simulink model "simulating astronaut"  (R2019b)
settings: Solver=ode45  StartTime=0.0  StopTime=600  FixedStep=.001  MaxStep=.01  MinStep=.001  RelTol=1e-3
values from neighbouring files (symbols this model uses):
  cmw_kPa = 0.0980665    [simulating astronaut.m]
  D = [1e-3 1e-2 0.545e-4]    [simulating astronaut.m]
  dc_metabool = [-0.250 0.200 0]/60    [simulating astronaut.m]
  dV_CO = 5/60    (= 0.0833333333333)    [simulating astronaut.m]
  f_alv_init = [0.154 0.0451 0.79 ]    [simulating astronaut.m]
  f_LW_init = [0.174 0.0291 0.79]    [simulating astronaut.m]
  Hbx_PA_init = [2.44 6.560 ]*1e-3    [simulating astronaut.m]
  Hbx_PC_init = [.564 8.436 ]*1e-3    [simulating astronaut.m]
  Hbx_SA_init = [.520 8.480 ]*1e-3    [simulating astronaut.m]
  Hbx_SC_init = [2.44 6.560 ]*1e-3    [simulating astronaut.m]
  k = 25.45    [simulating astronaut.m]
  P_LWO_EE = 5    [simulating astronaut.m]
  P_LWO_insp = 10    [simulating astronaut.m]
  p_O2_grenswaarde = 16    [simulating astronaut.m]
  p_PA_init = [4.34 11.3 56]    [simulating astronaut.m]
  p_PC_init = [6.92 3.45 55.7]    [simulating astronaut.m]
  p_SA_init = [7.11 3.26 56.4]    [simulating astronaut.m]
  p_SC_init = [4.34 11.3 56]    [simulating astronaut.m]
  p_weefsel_init = [4.33 11.3 56]    [simulating astronaut.m]
  period = 6    [simulating astronaut.m]
  pulse_width = 35    [simulating astronaut.m]
  R = [R_LW R_alv]    [simulating astronaut.m]
  s = [2.4e-4 5e-3 1.23e-4]    [simulating astronaut.m]
  t_left = 10    [simulating astronaut.m]
  t_right = 40    [simulating astronaut.m]
  V_init = [0.82 3.28]    [simulating astronaut.m]
  V_PC = .08    (= 0.08)    [simulating astronaut.m]
  V_SC = 0.250    (= 0.25)    [simulating astronaut.m]
  V_w = 5    [simulating astronaut.m]
  x_alv = [0.001 2 2.75 0.8]    [simulating astronaut.m]
  x_LW = [0.001 8 11 0.2]    [simulating astronaut.m]
  x_TW = [-240 -2.3 5 4.6]    [simulating astronaut.m]
settings Model: Creator=psomhorst  LastModifiedBy=Pruijt
settings DebuggingCC: ArithmeticOperatorsInVariantConditions=warning
settings SFSimCC: CustomCodeUndefinedFunction=UseInterfaceOnly

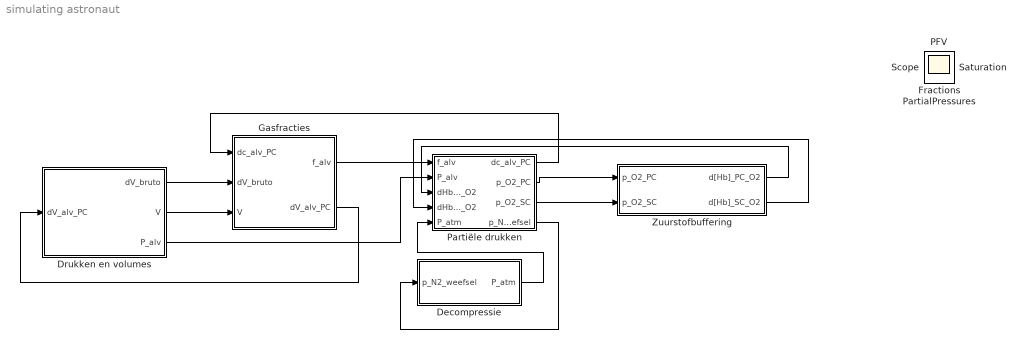
== system simulating astronaut ==
  "Decompressie " : Subsystem
  Drukken en volumes : Subsystem
  Gasfracties : Subsystem
  Partiële drukken : Subsystem
  "Zuurstofbuffering " : Subsystem
  Fractions : Scope
  PFV : Scope
  PartialPressures : Scope
  Saturation : Scope
  Scope : Scope
  wires:
  Drukken en volumes/1(dV_bruto) -> Gasfracties/2(dV_bruto)
  Drukken en volumes/2(V) -> Gasfracties/3(V)
  Gasfracties/2(dV_alv_PC) -> Drukken en volumes/1(dV_alv_PC)
  Gasfracties/1(f_alv) -> Partiële drukken/1(f_alv)
  Drukken en volumes/3(P_alv) -> Partiële drukken/2(P_alv)
  Partiële drukken/1(dc_alv_PC) -> Gasfracties/1(dc_alv_PC)
  Partiële drukken/2(p_O2_PC) -> "Zuurstofbuffering "/1(p_O2_PC)
  "Zuurstofbuffering "/1(d[Hb]_PC_O2) -> Partiële drukken/3(dHb_PC_O2)
  "Zuurstofbuffering "/2(d[Hb]_SC_O2) -> Partiële drukken/4(dHb_SC_O2)
  "Decompressie "/1("P_atm ") -> Partiële drukken/5("P_atm ")
  Partiële drukken/4("p_N2_weefsel ") -> "Decompressie "/1("p_N2_weefsel ")
  Partiële drukken/3(p_O2_SC) -> "Zuurstofbuffering "/2(p_O2_SC)

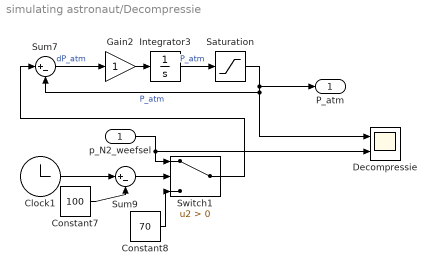
== system simulating astronaut/Decompressie  ==
  "p_N2_weefsel " : Inport
  Clock1 : Clock
  Constant7 : Constant  Value=100
  Constant8 : Constant  Value=70
  "Decompressie " : Scope  NumInputPorts=2
  Gain2 : Gain
  Integrator3 : Integrator  InitialCondition=70
  Saturation : Saturate  UpperLimit=71  LowerLimit=30
  Sum7 : Sum  Inputs=|+-
  Sum9 : Sum  Inputs=|+-
  Switch1 : Switch  Criteria=u2 > Threshold
  "P_atm " : Outport
  wires:
  Gain2/1 -> Integrator3/1
  Sum7/1 -> Gain2/1  "dP_atm"
  Integrator3/1 -> Saturation/1  "P_atm"
  Saturation/1 -> "Decompressie "/1, Sum7/2, "P_atm "/1  "P_atm"
  Constant7/1 -> Sum9/2
  Clock1/1 -> Sum9/1
  Sum9/1 -> Switch1/2
  "p_N2_weefsel "/1 -> "Decompressie "/2, Switch1/1
  Constant8/1 -> Switch1/3
  Switch1/1 -> Sum7/1

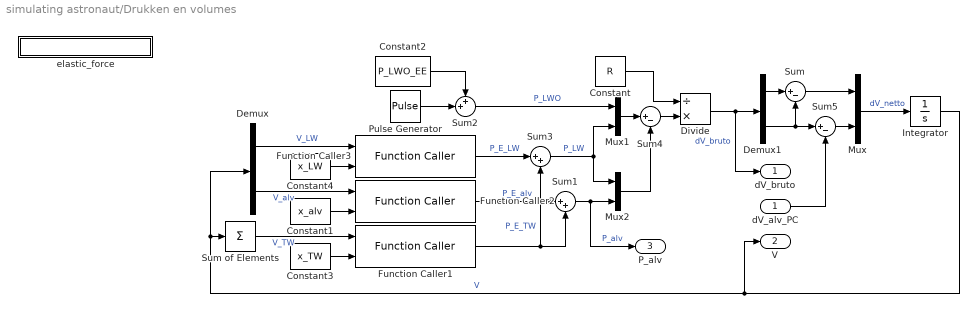
== system simulating astronaut/Drukken en volumes ==
  dV_alv_PC : Inport
  Constant : Constant  Value=R
  Constant1 : Constant  Value=x_alv
  Constant2 : Constant  Value=P_LWO_EE
  Constant3 : Constant  Value=x_TW
  Constant4 : Constant  Value=x_LW
  Demux : Demux  Outputs=2
  Demux1 : Demux  Outputs=2
  Divide : Product  Inputs=/*
  Function Caller1 : FunctionCaller  FunctionPrototype=P_E = elastic_force(V,x)  InputArgumentSpecifications=<Enter example>  OutputArgumentSpecifications=<Enter example>
  Function Caller2 : FunctionCaller  FunctionPrototype=P_E = elastic_force(V,x)  InputArgumentSpecifications=<Enter example>  OutputArgumentSpecifications=<Enter example>
  Function Caller3 : FunctionCaller  FunctionPrototype=P_E = elastic_force(V,x)  InputArgumentSpecifications=<Enter example>  OutputArgumentSpecifications=<Enter example>
  Integrator : Integrator  InitialCondition=V_init
  Mux : Mux  Inputs=2
  Mux1 : Mux  Inputs=2
  Mux2 : Mux  Inputs=2
  Pulse Generator : DiscretePulseGenerator  PulseType=Time based  Amplitude=P_LWO_insp  Period=period  PulseWidth=pulse_width
  Sum : Sum  Inputs=|+-
  Sum of Elements : Sum  Inputs=+
  Sum1 : Sum  Inputs=|++
  Sum2 : Sum  Inputs=++|
  Sum3 : Sum  Inputs=|++
  Sum4 : Sum  Inputs=|+-
  Sum5 : Sum  Inputs=|+-
  elastic_force : Subsystem  TreatAsAtomicUnit=on
  dV_bruto : Outport
  V : Outport  Port=2
  P_alv : Outport  Port=3
  wires:
  Mux2/1 -> Sum4/2
  Sum1/1 -> P_alv/1, Mux2/2  "P_alv"
  Demux/1 -> Function Caller3/1  "V_LW"
  Sum2/1 -> Mux1/1  "P_LWO"
  Mux1/1 -> Sum4/1
  Sum3/1 -> Mux2/1, Mux1/2  "P_LW"
  Demux1/1 -> Sum/1
  Function Caller3/1 -> Sum3/1  "P_E_LW"
  Function Caller2/1 -> Sum1/1  "P_E_alv"
  Sum of Elements/1 -> Function Caller1/1  "V_TW"
  Constant2/1 -> Sum2/1
  Pulse Generator/1 -> Sum2/2
  Constant4/1 -> Function Caller3/2
  Divide/1 -> Demux1/1, dV_bruto/1  "dV_bruto"
  Demux/2 -> Function Caller2/1  "V_alv"
  Integrator/1 -> Demux/1, Sum of Elements/1, V/1  "V"
  Sum/1 -> Mux/1
  Sum4/1 -> Divide/2
  Mux/1 -> Integrator/1  "dV_netto"
  Function Caller1/1 -> Sum1/2, Sum3/2  "P_E_TW"
  Constant1/1 -> Function Caller2/2
  Constant3/1 -> Function Caller1/2
  Demux1/2 -> Sum5/1, Sum/2
  Constant/1 -> Divide/1
  Sum5/1 -> Mux/2
  dV_alv_PC/1 -> Sum5/2

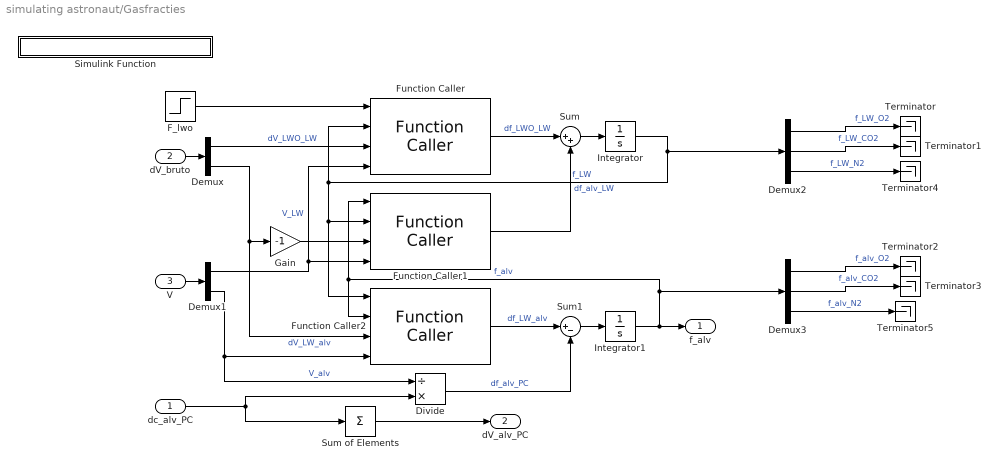
== system simulating astronaut/Gasfracties ==
  dc_alv_PC : Inport
  dV_bruto : Inport  Port=2
  V : Inport  Port=3
  Demux : Demux  Outputs=2
  Demux1 : Demux  Outputs=2
  Demux2 : Demux  Outputs=3
  Demux3 : Demux  Outputs=3
  Divide : Product  Inputs=/*
  "F_lwo " : Step  Time=100  Before=[.21 0 .79]  After=[1 0 0]  SampleTime=0
  Function Caller : FunctionCaller  FunctionPrototype=df = fraction_change(f1,f2,dV,V)  InputArgumentSpecifications=<Enter example>  OutputArgumentSpecifications=<Enter example>
  Function Caller1 : FunctionCaller  FunctionPrototype=df = fraction_change(f1,f2,dV,V)  InputArgumentSpecifications=<Enter example>  OutputArgumentSpecifications=<Enter example>
  Function Caller2 : FunctionCaller  FunctionPrototype=df = fraction_change(f1,f2,dV,V)  InputArgumentSpecifications=<Enter example>  OutputArgumentSpecifications=<Enter example>
  Gain : Gain  Gain=-1
  Integrator : Integrator  InitialCondition=f_LW_init
  Integrator1 : Integrator  InitialCondition=f_alv_init
  Simulink Function : Subsystem  TreatAsAtomicUnit=on
  Sum : Sum  Inputs=|++
  Sum of Elements : Sum  Inputs=+
  Sum1 : Sum  Inputs=|+-
  Terminator{,1..5} (6 alike) : Terminator
  f_alv : Outport
  dV_alv_PC : Outport  Port=2
  wires:
  Integrator/1 -> Function Caller2/1, Function Caller1/2, Function Caller/2, Demux2/1  "f_LW"
  Integrator1/1 -> f_alv/1, Function Caller2/2, Function Caller1/1, Demux3/1  "f_alv"
  "F_lwo "/1 -> Function Caller/1
  Gain/1 -> Function Caller1/3
  dV_bruto/1 -> Demux/1
  V/1 -> Demux1/1
  Demux1/1 -> Function Caller/4, Function Caller1/4  "V_LW"
  Demux1/2 -> Divide/1, Function Caller2/4  "V_alv"
  Demux/1 -> Function Caller/3  "dV_LWO_LW"
  Demux/2 -> Function Caller2/3, Gain/1  "dV_LW_alv"
  Function Caller/1 -> Sum/1  "df_LWO_LW"
  Function Caller1/1 -> Sum/2  "df_alv_LW"
  Sum/1 -> Integrator/1
  dc_alv_PC/1 -> Divide/2, Sum of Elements/1
  Sum1/1 -> Integrator1/1
  Function Caller2/1 -> Sum1/1  "df_LW_alv"
  Divide/1 -> Sum1/2  "df_alv_PC"
  Demux3/2 -> Terminator3/1  "f_alv_CO2"
  Demux2/1 -> Terminator/1  "f_LW_O2"
  Demux2/2 -> Terminator1/1  "f_LW_CO2"
  Demux3/1 -> Terminator2/1  "f_alv_O2"
  Sum of Elements/1 -> dV_alv_PC/1
  Demux2/3 -> Terminator4/1  "f_LW_N2"
  Demux3/3 -> Terminator5/1  "f_alv_N2"

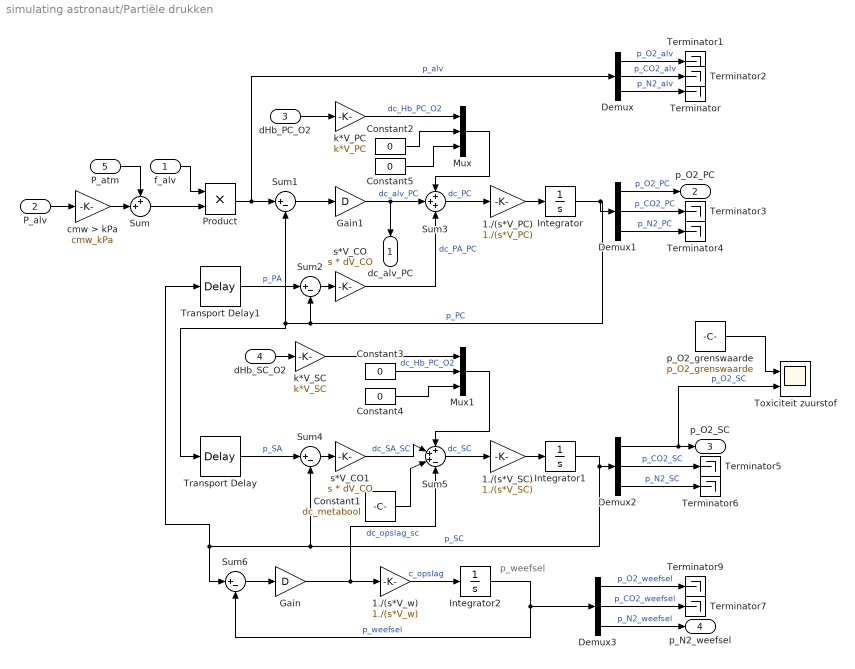
== system simulating astronaut/Partiële drukken ==
  note: p_weefsel
  f_alv : Inport
  P_alv : Inport  Port=2
  dHb_PC_O2 : Inport  Port=3
  dHb_SC_O2 : Inport  Port=4
  "P_atm " : Inport  Port=5
  1./(s*V_PC) : Gain  Gain=1./(s*V_PC)
  1./(s*V_SC) : Gain  Gain=1./(s*V_SC)
  1./(s*V_w) : Gain  Gain=1./(s*V_w)
  Constant1 : Constant  Value=dc_metabool
  Constant{2..5} (4 alike) : Constant  Value=0
  Demux{,1..3} (4 alike) : Demux  Outputs=3
  Gain : Gain  Gain=D
  Gain1 : Gain  Gain=D
  Integrator : Integrator  InitialCondition=p_PC_init
  Integrator1 : Integrator  InitialCondition=p_SC_init
  Integrator2 : Integrator  InitialCondition=p_weefsel_init
  Mux : Mux  Inputs=3
  Mux1 : Mux  Inputs=3
  Product : Product
  Sum : Sum  Inputs=++|
  Sum{1..2,4,6} (4 alike) : Sum  Inputs=|+-
  Sum3 : Sum  Inputs=+++
  Sum5 : Sum  Inputs=+++-
  Terminator{,1..7,9} (9 alike) : Terminator
  "Toxiciteit zuurstof " : Scope  NumInputPorts=2
  Transport Delay : TransportDelay  DelayTime=t_left  InitialOutput=p_SA_init  BufferSize=10240
  Transport Delay1 : TransportDelay  DelayTime=t_right  InitialOutput=p_PA_init  BufferSize=40960
  cmw > kPa : Gain  Gain=cmw_kPa
  k*V_PC : Gain  Gain=k*V_PC
  k*V_SC : Gain  Gain=k*V_SC
  "p_O2_grenswaarde " : Constant  Value=p_O2_grenswaarde
  s*V_CO : Gain  Gain=s * dV_CO
  s*V_CO1 : Gain  Gain=s * dV_CO
  dc_alv_PC : Outport
  p_O2_PC : Outport  Port=2
  p_O2_SC : Outport  Port=3
  "p_N2_weefsel " : Outport  Port=4
  wires:
  f_alv/1 -> Product/1
  Product/1 -> Demux/1, Sum1/1  "p_alv"
  Integrator/1 -> Transport Delay/1, Sum1/2, Sum2/2, Demux1/1  "p_PC"
  Sum1/1 -> Gain1/1
  Gain1/1 -> Sum3/2, dc_alv_PC/1  "dc_alv_PC"
  1./(s*V_PC)/1 -> Integrator/1
  Demux/1 -> Terminator1/1  "p_O2_alv"
  Demux1/1 -> p_O2_PC/1  "p_O2_PC"
  Demux/2 -> Terminator2/1  "p_CO2_alv"
  Demux1/2 -> Terminator3/1  "p_CO2_PC"
  Transport Delay1/1 -> Sum2/1  "p_PA"
  Sum3/1 -> 1./(s*V_PC)/1  "dc_PC"
  Sum2/1 -> s*V_CO/1
  Transport Delay/1 -> Sum4/1  "p_SA"
  Sum4/1 -> s*V_CO1/1
  1./(s*V_SC)/1 -> Integrator1/1
  Demux2/2 -> Terminator5/1  "p_CO2_SC"
  Demux2/1 -> p_O2_SC/1, "Toxiciteit zuurstof "/2  "p_O2_SC"
  Integrator1/1 -> Sum4/2, Sum6/1, Transport Delay1/1, Demux2/1  "p_SC"
  Sum5/1 -> 1./(s*V_SC)/1  "dc_SC"
  s*V_CO1/1 -> Sum5/2  "dc_SA_SC"
  dHb_SC_O2/1 -> k*V_SC/1
  dHb_PC_O2/1 -> k*V_PC/1
  s*V_CO/1 -> Sum3/3  "dc_PA_PC"
  k*V_PC/1 -> Mux/1  "dc_Hb_PC_O2"
  Mux/1 -> Sum3/1
  Constant2/1 -> Mux/2
  Constant3/1 -> Mux1/2
  k*V_SC/1 -> Mux1/1  "dc_Hb_PC_O2"
  Mux1/1 -> Sum5/1
  Demux/3 -> Terminator/1  "p_N2_alv"
  Demux1/3 -> Terminator4/1  "p_N2_PC"
  Demux2/3 -> Terminator6/1  "p_N2_SC"
  Constant4/1 -> Mux1/3
  Constant5/1 -> Mux/3
  Constant1/1 -> Sum5/3
  Sum6/1 -> Gain/1
  1./(s*V_w)/1 -> Integrator2/1  "c_opslag"
  Gain/1 -> 1./(s*V_w)/1, Sum5/4  "dc_opslag_sc"
  P_alv/1 -> cmw > kPa/1
  cmw > kPa/1 -> Sum/2
  Sum/1 -> Product/2
  Integrator2/1 -> Sum6/2, Demux3/1  "p_weefsel"
  Demux3/3 -> "p_N2_weefsel "/1  "p_N2_weefsel"
  Demux3/1 -> Terminator9/1  "p_O2_weefsel"
  Demux3/2 -> Terminator7/1  "p_CO2_weefsel"
  "p_O2_grenswaarde "/1 -> "Toxiciteit zuurstof "/1
  "P_atm "/1 -> Sum/1

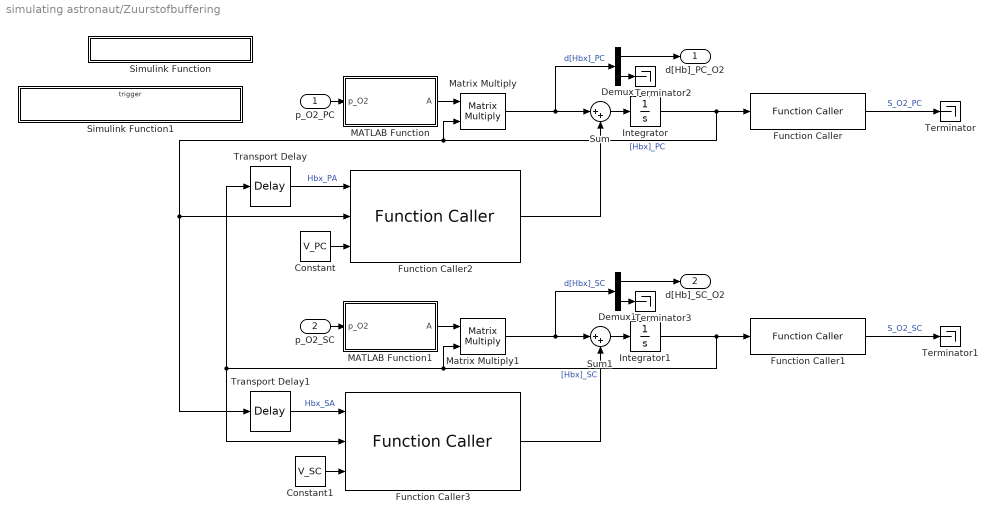
== system simulating astronaut/Zuurstofbuffering  ==
  p_O2_PC : Inport
  p_O2_SC : Inport  Port=2
  Constant : Constant  Value=V_PC
  Constant1 : Constant  Value=V_SC
  Demux : Demux  Outputs=2
  Demux1 : Demux  Outputs=2
  Function Caller : FunctionCaller  FunctionPrototype=S_O2 = saturation(Hbx)  InputArgumentSpecifications=<Enter example>  OutputArgumentSpecifications=<Enter example>
  Function Caller1 : FunctionCaller  FunctionPrototype=S_O2 = saturation(Hbx)  InputArgumentSpecifications=<Enter example>  OutputArgumentSpecifications=<Enter example>
  Function Caller2 : FunctionCaller  FunctionPrototype=dHbx = Hb_circulation(Hbx_in,Hbx_out,V)  InputArgumentSpecifications=<Enter example>  OutputArgumentSpecifications=<Enter example>
  Function Caller3 : FunctionCaller  FunctionPrototype=dHbx = Hb_circulation(Hbx_in,Hbx_out,V)  InputArgumentSpecifications=<Enter example>  OutputArgumentSpecifications=<Enter example>
  Integrator : Integrator  InitialCondition=Hbx_PC_init
  Integrator1 : Integrator  InitialCondition=Hbx_SC_init
  MATLAB Function : MATLAB Function  TreatAsAtomicUnit=on
  MATLAB Function1 : MATLAB Function  TreatAsAtomicUnit=on
  Matrix Multiply : Product  Multiplication=Matrix(*)
  Matrix Multiply1 : Product  Multiplication=Matrix(*)
  Simulink Function : Subsystem  TreatAsAtomicUnit=on
  Simulink Function1 : Subsystem  TreatAsAtomicUnit=on
  Sum : Sum  Inputs=|++
  Sum1 : Sum  Inputs=|++
  Terminator{,1..3} (4 alike) : Terminator
  Transport Delay : TransportDelay  DelayTime=t_right  InitialOutput=Hbx_PA_init  BufferSize=40960
  Transport Delay1 : TransportDelay  DelayTime=t_left  InitialOutput=Hbx_SA_init  BufferSize=10240
  d[Hb]_PC_O2 : Outport
  d[Hb]_SC_O2 : Outport  Port=2
  wires:
  Integrator/1 -> Function Caller/1, Function Caller2/2, Transport Delay1/1, Matrix Multiply/2  "[Hbx]_PC"
  MATLAB Function/1(A) -> Matrix Multiply/1
  p_O2_PC/1 -> MATLAB Function/1(p_O2)
  Matrix Multiply/1 -> Sum/1, Demux/1  "d[Hbx]_PC"
  Function Caller/1 -> Terminator/1  "S_O2_PC"
  Integrator1/1 -> Function Caller1/1, Transport Delay/1, Function Caller3/2, Matrix Multiply1/2  "[Hbx]_SC"
  MATLAB Function1/1(A) -> Matrix Multiply1/1
  p_O2_SC/1 -> MATLAB Function1/1(p_O2)
  Function Caller1/1 -> Terminator1/1  "S_O2_SC"
  Demux/1 -> d[Hb]_PC_O2/1
  Demux/2 -> Terminator2/1
  Demux1/1 -> d[Hb]_SC_O2/1
  Matrix Multiply1/1 -> Sum1/1, Demux1/1  "d[Hbx]_SC"
  Demux1/2 -> Terminator3/1
  Sum/1 -> Integrator/1
  Function Caller2/1 -> Sum/2
  Sum1/1 -> Integrator1/1
  Function Caller3/1 -> Sum1/2
  Constant/1 -> Function Caller2/3
  Constant1/1 -> Function Caller3/3
  Transport Delay/1 -> Function Caller2/1  "Hbx_PA"
  Transport Delay1/1 -> Function Caller3/1  "Hbx_SA"

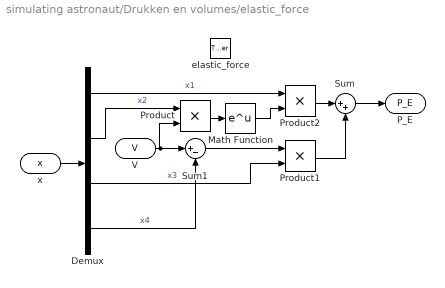
== system simulating astronaut/Drukken en volumes/elastic_force ==
  elastic_force : TriggerPort  TriggerType=function-call  IsSimulinkFunction=on  FunctionName=elastic_force  FunctionVisibility=scoped  VariantControl=(inherit)
  Demux : Demux
  Math Function : Math  SaturateOnIntegerOverflow=on
  Product : Product
  Product1 : Product
  Product2 : Product
  Sum : Sum  Inputs=|++
  Sum1 : Sum  Inputs=|+-
  V : ArgIn  DisableCoverage=on  ArgumentName=V
  x : ArgIn  Port=2  PortDimensions=4  ArgumentName=x
  P_E : ArgOut  DisableCoverage=on  ArgumentName=P_E
  wires:
  Product/1 -> Math Function/1
  Sum/1 -> P_E/1
  Product1/1 -> Sum/2
  V/1 -> Product/2, Sum1/1
  x/1 -> Demux/1
  Demux/1 -> Product2/1  "x1"
  Math Function/1 -> Product2/2
  Sum1/1 -> Product1/1
  Product2/1 -> Sum/1
  Demux/2 -> Product/1  "x2"
  Demux/3 -> Product1/2  "x3"
  Demux/4 -> Sum1/2  "x4"

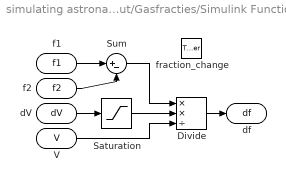
== system simulating astronaut/Gasfracties/Simulink Function ==
  fraction_change : TriggerPort  TriggerType=function-call  IsSimulinkFunction=on  FunctionName=fraction_change  FunctionVisibility=scoped  VariantControl=(inherit)
  Divide : Product  Inputs=**/
  Saturation : Saturate  UpperLimit=inf  LowerLimit=0
  Sum : Sum  Inputs=|+-
  f1 : ArgIn  DisableCoverage=on  PortDimensions=3  ArgumentName=f1
  f2 : ArgIn  Port=2  PortDimensions=3  ArgumentName=f2
  dV : ArgIn  Port=3  ArgumentName=dV
  V : ArgIn  Port=4  ArgumentName=V
  df : ArgOut  DisableCoverage=on  PortDimensions=3  ArgumentName=df
  wires:
  f1/1 -> Sum/1
  f2/1 -> Sum/2
  dV/1 -> Saturation/1
  Saturation/1 -> Divide/2
  Sum/1 -> Divide/1
  V/1 -> Divide/3
  Divide/1 -> df/1

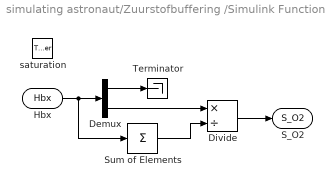
== system simulating astronaut/Zuurstofbuffering /Simulink Function ==
  saturation : TriggerPort  TriggerType=function-call  IsSimulinkFunction=on  FunctionName=saturation  FunctionVisibility=scoped  VariantControl=(inherit)
  Demux : Demux  Outputs=2
  Divide : Product  Inputs=*/
  Sum of Elements : Sum  Inputs=+
  Terminator : Terminator
  Hbx : ArgIn  DisableCoverage=on  PortDimensions=2  ArgumentName=Hbx
  S_O2 : ArgOut  DisableCoverage=on  ArgumentName=S_O2
  wires:
  Hbx/1 -> Sum of Elements/1, Demux/1
  Demux/1 -> Terminator/1
  Demux/2 -> Divide/1
  Sum of Elements/1 -> Divide/2
  Divide/1 -> S_O2/1

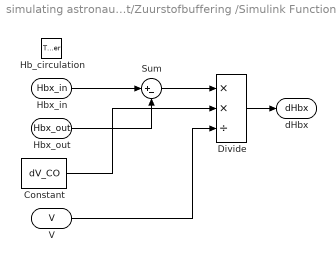
== system simulating astronaut/Zuurstofbuffering /Simulink Function1 ==
  Hb_circulation : TriggerPort  TriggerType=function-call  IsSimulinkFunction=on  FunctionName=Hb_circulation  FunctionVisibility=scoped  VariantControl=(inherit)
  Constant : Constant  Value=dV_CO
  Divide : Product  Inputs=**/
  Sum : Sum  Inputs=|+-
  Hbx_in : ArgIn  DisableCoverage=on  PortDimensions=2  ArgumentName=Hbx_in
  Hbx_out : ArgIn  Port=2  PortDimensions=2  ArgumentName=Hbx_out
  V : ArgIn  Port=3  ArgumentName=V
  dHbx : ArgOut  DisableCoverage=on  PortDimensions=2  ArgumentName=dHbx
  wires:
  Hbx_in/1 -> Sum/1
  Hbx_out/1 -> Sum/2
  Sum/1 -> Divide/1
  Constant/1 -> Divide/2
  V/1 -> Divide/3
  Divide/1 -> dHbx/1

== matlab function simulating astronaut/Zuurstofbuffering /MATLAB Function1 ==
  data: p_O2 input; A output
function A = get_matrix(p_O2)

ka = 0.8 * p_O2;
kd = 37.65 * p_O2^-1.87;

A = [-ka kd; ka -kd];

== matlab function simulating astronaut/Zuurstofbuffering /MATLAB Function ==
  data: p_O2 input; A output
function A = get_matrix(p_O2)

ka = 0.8 * p_O2;
kd = 37.65 * p_O2^-1.87;

A = [-ka kd; ka -kd];
